simulink library "libex"  (R2021b)
settings: Solver=VariableStepAuto  StartTime=0.0  StopTime=10.0  RelTol=1e-3
libraries: $bdroot x1
settings Model: Creator=fredric  LastModifiedBy=fredric

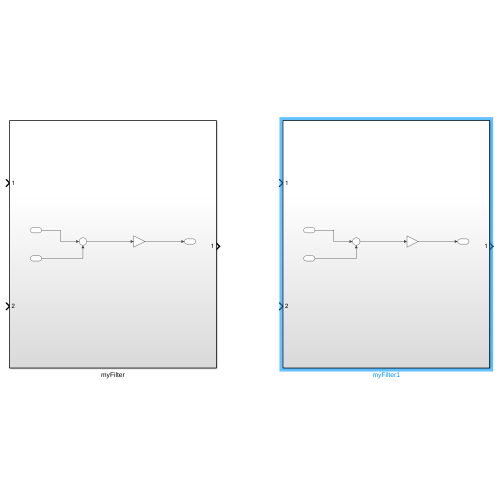
[thumbnail: Simulink's stored preview of the top-level diagram]
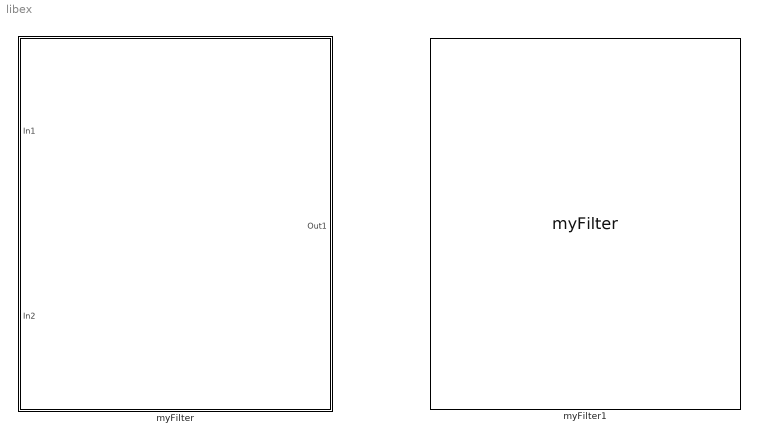
== system libex ==
  myFilter : Subsystem
  myFilter1 : $bdroot/myFilter  SystemSampleTime=-1  VariantActivationTime=update diagram  Latency=0  AutoFrameSizeCalculation=off

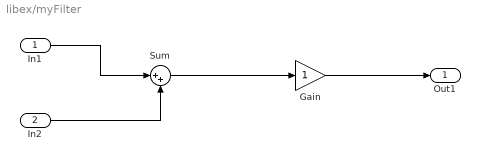
== system libex/myFilter ==
  In1 : Inport
  In2 : Inport  Port=2
  Gain : Gain
  Sum : Sum  Inputs=|++
  Out1 : Outport
  wires:
  Gain/1 -> Out1/1
  In2/1 -> Sum/2
  In1/1 -> Sum/1
  Sum/1 -> Gain/1
